simulink model "FlightSimulation"  (R2025a)
settings: Solver=ode4  StartTime=0.0  StopTime=Inf  FixedStep=time.dt  MaxStep=0.001  RelTol=1e-3
values from neighbouring files (symbols this model uses):
  AeroModel = init_IREC2025_CFDModel()    [RunSimulink.m]
  const = setupConstants()    [RunSimulink.m]
  kfConsts = getKfConsts()    [RunSimulink.m]
  kfErrInds = getErrorKfInds()    [RunSimulink.m]
  kfInds = getKfInds()    [RunSimulink.m]
  kfParams = initNavParams(kins)    [RunSimulink.m]
  kins = HPRC_RocketKinematics()    [RunSimulink.m]
  launchLLA = [launchLat, launchLon, launchAlt]    [RunSimulink.m]
  MotorModel = initMotorModel()    [RunSimulink.m]
  w_ib_x = 1e-10    [RunSimulink.m]
  w_ib_y = 1e-10    [RunSimulink.m]
  w_ib_z = 1e-10    [RunSimulink.m]
undefined symbols (not defined in the file or in its folder): Earth, F, fractalcoef, Light, MIL, Receive, Send, Sim3dSensor, simCfg, time, WGS84, WMM2020
libraries: simulink x6, aerolibatmos2 x5, aerolibfltsims x2, sim3dlib x2, aerolibsim3d x2, mspsensorlib x1, aerolibnav x1, aerolibgravity2 x1, aerolib6dof2 x1, aerolibwind2 x1, simulink_extras x1, matrix_library x1
(part 1 of 2)
settings Model: Creator=Blind  LastModifiedBy=Blind

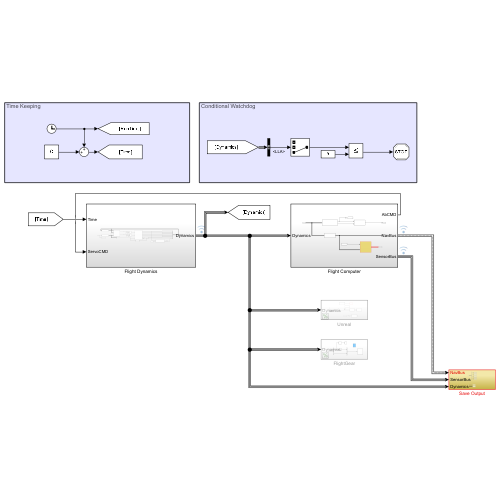
[thumbnail: Simulink's stored preview of the top-level diagram]
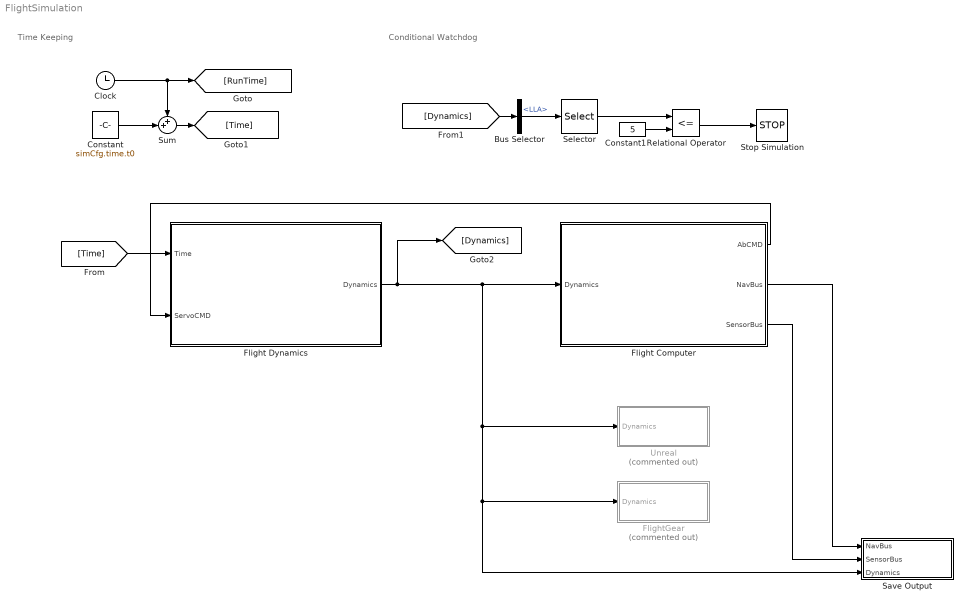
== system FlightSimulation ==
  note: Time Keeping
  note: Conditional Watchdog
  Bus Selector : BusSelector  OutputSignals=LLA
  Clock : Clock
  Constant : Constant  Value=simCfg.time.t0
  Constant1 : Constant  Value=5
  Flight Computer : Subsystem
  Flight Dynamics : Subsystem
  FlightGear : Subsystem  Commented=on
  Relational Operator : RelationalOperator  Operator=<=  OutDataTypeStr=boolean  RndMeth=Simplest  InputSameDT=off
  Save Output : Subsystem
  Selector : Selector  InputPortWidth=3  IndexOptions=Index vector (dialog)  Indices=3  OutputSizes=1
  Stop Simulation : Stop
  Sum : Sum  Inputs=++|
  Unreal : Subsystem  Commented=on
  wires:
  Clock/1 -> Sum/1, [RunTime]
  Constant/1 -> Sum/2
  Sum/1 -> [Time]
  [Time] -> Flight Dynamics/1(Time)
  Flight Dynamics/1(Dynamics) -> Flight Computer/1(Dynamics), Unreal/1(Dynamics), Save Output/3(Dynamics), FlightGear/1(Dynamics), [Dynamics]
  [Dynamics] -> Bus Selector/1
  Bus Selector/1 -> Selector/1  "<LLA>"
  Selector/1 -> Relational Operator/1
  Constant1/1 -> Relational Operator/2
  Relational Operator/1 -> Stop Simulation/1
  Flight Computer/1(AbCMD) -> Flight Dynamics/2(ServoCMD)
  Flight Computer/2(NavBus) -> Save Output/1(NavBus)
  Flight Computer/3(SensorBus) -> Save Output/2(SensorBus)

== system FlightSimulation/Flight Computer ==
  Dynamics : Inport
  Navigator : Subsystem  TreatAsAtomicUnit=on  SystemSampleTime=time.navDt
  Sensor Bus : Subsystem  TreatAsAtomicUnit=on
  State Machine : Subsystem
  Subsystem : Subsystem
  AbCMD : Outport
  NavBus : Outport  Port=2
  SensorBus : Outport  Port=3
  wires:
  Dynamics/1 -> Sensor Bus/1(Dynamics), State Machine/1(Dynamics)
  State Machine/1(State) -> [State], Subsystem/1(State)
  Subsystem/1(AbCMD) -> AbCMD/1
  State Machine/2(Guid) -> Subsystem/2(Guid)
  Sensor Bus/1(SensorBus) -> SensorBus/1, Navigator/2(SensorBus)
  Navigator/1(NavBus) -> NavBus/1
  [State] -> Navigator/1(State)

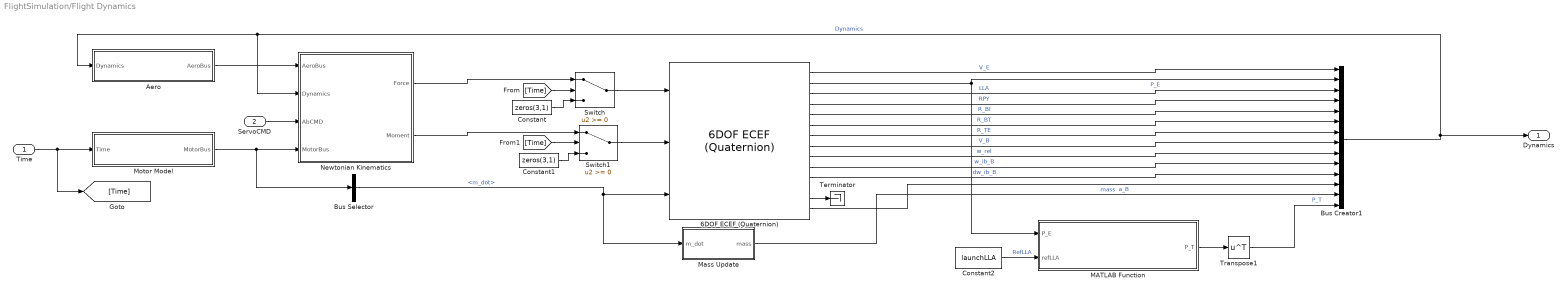
== system FlightSimulation/Flight Dynamics ==
  Time : Inport
  ServoCMD : Inport  Port=2
  6DOF ECEF (Quaternion) : aerolib6dof2/6DOF ECEF (Quaternion)  units=Metric (MKS)  mtype=Simple Variable  xg_0=launchLLA  Vm_0=V_0_B  eul_0=eul_0  pm_0=[w_ib_x; w_ib_y; w_ib_z]  mass_0=kins.m_0 + MotorModel.emptyWt + MotorModel.propWt  mass_e=kins.m_0 + MotorModel.emptyWt  mass_f=kins.m_0 + MotorModel.emptyWt + MotorModel.propWt  inertia=eye(3)  inertia_e=kins.I_empty  inertia_f=kins.I_full  vre_flag=off  abi_flag=on  ptype=Earth (WGS84)  R=6378137  F=1/298.257223563  w_E=7292115e-11  angle_in=Internal  LPM0=0  quat_statename=''  pm_statename=''  Vm_statename=''  posfixedframe_statename=''  posinertial_statename=''  LPM_statename=''  mass_statename=''
  Aero : Subsystem
  Bus Creator1 : BusCreator  Inputs=14
  Bus Selector : BusSelector  OutputSignals=m_dot
  Constant : Constant  Value=zeros(3,1)
  Constant1 : Constant  Value=zeros(3,1)
  Constant2 : Constant  Value=launchLLA
  MATLAB Function : MATLAB Function  TreatAsAtomicUnit=on
  Mass Update : Subsystem
  Motor Model : Subsystem
  Newtonian Kinematics : Subsystem
  Switch : Switch  SaturateOnIntegerOverflow=off  InputSameDT=off
  Switch1 : Switch  SaturateOnIntegerOverflow=off  InputSameDT=off
  Terminator : Terminator
  Transpose1 : Math  Operator=transpose
  Dynamics : Outport
  wires:
  Motor Model/1(MotorBus) -> Newtonian Kinematics/4(MotorBus), Bus Selector/1
  Time/1 -> [Time], Motor Model/1(Time)
  Bus Creator1/1 -> Newtonian Kinematics/2(Dynamics), Aero/1(Dynamics), Dynamics/1  "Dynamics"
  Aero/1(AeroBus) -> Newtonian Kinematics/1(AeroBus)
  Bus Selector/1 -> Mass Update/1(m_dot), 6DOF ECEF (Quaternion)/3  "<m_dot>"
  6DOF ECEF (Quaternion)/1 -> Bus Creator1/1  "V_E"
  6DOF ECEF (Quaternion)/2 -> MATLAB Function/1(P_E), Bus Creator1/2  "P_E"
  6DOF ECEF (Quaternion)/4 -> Bus Creator1/4  "RPY"
  6DOF ECEF (Quaternion)/5 -> Bus Creator1/5  "R_BI"
  6DOF ECEF (Quaternion)/6 -> Bus Creator1/6  "R_BT"
  6DOF ECEF (Quaternion)/7 -> Bus Creator1/7  "R_TE"
  6DOF ECEF (Quaternion)/8 -> Bus Creator1/8  "V_B"
  6DOF ECEF (Quaternion)/10 -> Bus Creator1/10  "w_ib_B"
  6DOF ECEF (Quaternion)/11 -> Bus Creator1/11  "dw_ib_B"
  Mass Update/1(mass) -> Bus Creator1/13  "mass"
  6DOF ECEF (Quaternion)/3 -> Bus Creator1/3  "LLA"
  6DOF ECEF (Quaternion)/9 -> Bus Creator1/9  "w_rel"
  Newtonian Kinematics/1(Force) -> Switch/1
  [Time] -> Switch/2
  Constant/1 -> Switch/3
  Switch/1 -> 6DOF ECEF (Quaternion)/1
  [Time] -> Switch1/2
  Constant1/1 -> Switch1/3
  Newtonian Kinematics/2(Moment) -> Switch1/1
  Switch1/1 -> 6DOF ECEF (Quaternion)/2
  6DOF ECEF (Quaternion)/13 -> Terminator/1
  ServoCMD/1 -> Newtonian Kinematics/3(AbCMD)
  6DOF ECEF (Quaternion)/14 -> Bus Creator1/12  "a_B"
  MATLAB Function/1(P_T) -> Transpose1/1
  Constant2/1 -> MATLAB Function/2(refLLA)  "RefLLA"
  Transpose1/1 -> Bus Creator1/14  "P_T"

== system FlightSimulation/FlightGear ==
  Dynamics : Inport
  Bus Selector : BusSelector  OutputSignals=LLA,RPY
  FlightGear Preconfigured 6DoF Animation : aerolibfltsims/FlightGear Preconfigured 6DoF Animation  xFlightGearVersion=v2019.1  DestinationIpAddress=127.0.0.1  DestinationPort=5502  SampleTime=1/30  packetVersion=24
  Generate Run Script : aerolibfltsims/Generate Run Script  Architecture=Mac  dataFlow=Send-Receive  GeometryModelName=HPMR  AirportId=KORH  RunwayId=29  InitialAltitude=7224  InitialHeading=113  OffsetDistance=4.72  OffsetAzimuth=0  InstallScenery=on  DisableShaders=on  OriginAddress=127.0.0.1  DestinationPort=5502  OriginPort=5505  LocalAddress=127.0.0.1  OutputFileName=runfg.sh  FlightGearBaseDirectory=/Applications/FlightGear.app
  Scope : Scope
      settings: ActiveDisplayYMinimum=2705.45233  ActiveDisplayYMaximum=2716.52751
  Selector : Selector  InputPortWidth=3  IndexOptions=Index vector (dialog)  Indices=[2 1 3]  OutputSizes=1
  Selector1 : Selector  InputPortWidth=3  IndexOptions=Index vector (dialog)  Indices=3  OutputSizes=1
  Vector Concatenate : Concatenate
  wires:
  Dynamics/1 -> Bus Selector/1
  Bus Selector/2 -> Vector Concatenate/2  "<RPY>"
  Vector Concatenate/1 -> FlightGear Preconfigured 6DoF Animation/1
  Bus Selector/1 -> Selector1/1, Selector/1  "<LLA>"
  Selector/1 -> Vector Concatenate/1
  Selector1/1 -> Scope/1

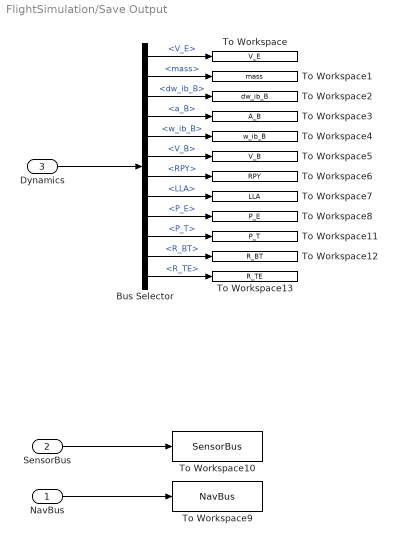
== system FlightSimulation/Save Output ==
  NavBus : Inport
  SensorBus : Inport  Port=2
  Dynamics : Inport  Port=3
  Bus Selector : BusSelector  OutputSignals=V_E,mass,dw_ib_B,a_B,w_ib_B,V_B,RPY,LLA,P_E,P_T,R_BT,R_TE
  To Workspace : ToWorkspace  VariableName=V_E  SaveFormat=Timeseries  SampleTime=-1
  To Workspace1 : ToWorkspace  VariableName=mass  SaveFormat=Timeseries  SampleTime=-1
  To Workspace10 : ToWorkspace  VariableName=SensorBus  SaveFormat=Timeseries  SampleTime=-1
  To Workspace11 : ToWorkspace  VariableName=P_T  SaveFormat=Timeseries  SampleTime=-1
  To Workspace12 : ToWorkspace  VariableName=R_BT  SaveFormat=Timeseries  SampleTime=-1
  To Workspace13 : ToWorkspace  VariableName=R_TE  SaveFormat=Timeseries  SampleTime=-1
  To Workspace2 : ToWorkspace  VariableName=dw_ib_B  SaveFormat=Timeseries  SampleTime=-1
  To Workspace3 : ToWorkspace  VariableName=A_B  SaveFormat=Timeseries  SampleTime=-1
  To Workspace4 : ToWorkspace  VariableName=w_ib_B  SaveFormat=Timeseries  SampleTime=-1
  To Workspace5 : ToWorkspace  VariableName=V_B  SaveFormat=Timeseries  SampleTime=-1
  To Workspace6 : ToWorkspace  VariableName=RPY  SaveFormat=Timeseries  SampleTime=-1
  To Workspace7 : ToWorkspace  VariableName=LLA  SaveFormat=Timeseries  SampleTime=-1
  To Workspace8 : ToWorkspace  VariableName=P_E  SaveFormat=Timeseries  SampleTime=-1
  To Workspace9 : ToWorkspace  VariableName=NavBus  SaveFormat=Timeseries  SampleTime=-1
  wires:
  Dynamics/1 -> Bus Selector/1
  Bus Selector/1 -> To Workspace/1  "<V_E>"
  Bus Selector/2 -> To Workspace1/1  "<mass>"
  Bus Selector/3 -> To Workspace2/1  "<dw_ib_B>"
  Bus Selector/4 -> To Workspace3/1  "<a_B>"
  Bus Selector/5 -> To Workspace4/1  "<w_ib_B>"
  Bus Selector/6 -> To Workspace5/1  "<V_B>"
  Bus Selector/7 -> To Workspace6/1  "<RPY>"
  Bus Selector/8 -> To Workspace7/1  "<LLA>"
  Bus Selector/9 -> To Workspace8/1  "<P_E>"
  NavBus/1 -> To Workspace9/1
  SensorBus/1 -> To Workspace10/1
  Bus Selector/10 -> To Workspace11/1  "<P_T>"
  Bus Selector/11 -> To Workspace12/1  "<R_BT>"
  Bus Selector/12 -> To Workspace13/1  "<R_TE>"

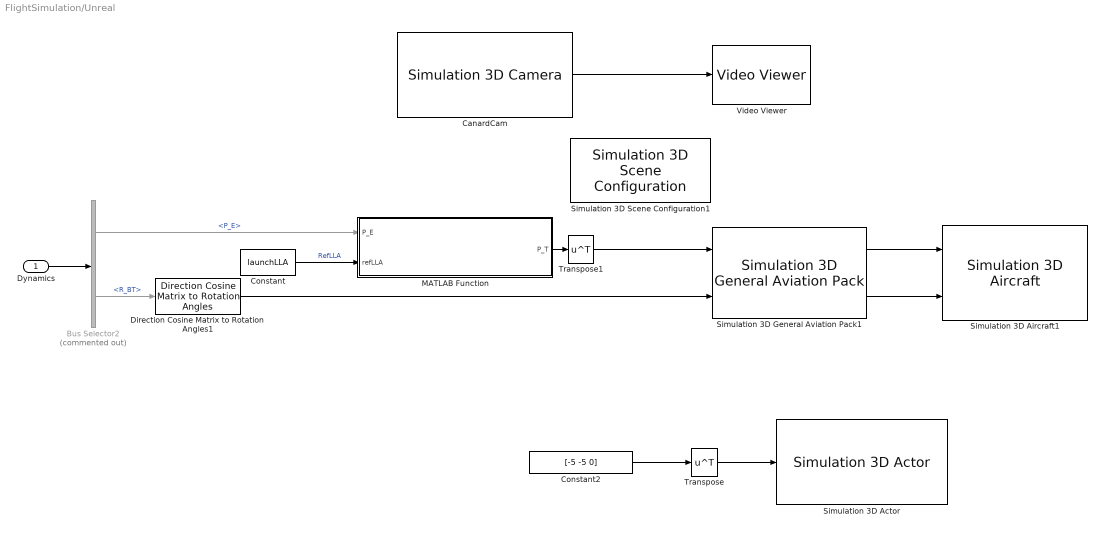
== system FlightSimulation/Unreal ==
  Dynamics : Inport
  Bus Selector2 : BusSelector  Commented=on  OutputSignals=P_E,R_BT
  CanardCam : sim3dcameralib/Simulation 3D Camera  Priority=1  sensorTag=Sim3dSensor�  sensorId=1  sensorName=Sim3dSensor�  vehTagList={'MissileNED';'Scene Origin';'Sim3dActor1'}  vehTag=MissileNED  CoordinateSystem=ISO8855  mountLoc=Origin  offsetFlag=on  tmountOffset=[1, 0.14, 0]  extTmount=off  rmountOffset=[0, 0, 180]  extRmount=off  FocalLength=[1109, 1109]  OpticalCenter=[640, 360]  ImageSize=[720, 1280]  RadialDistortion=[0, 0]  TangentialDistortion=[0, 0]  SensorSkew=0  VisualizeFieldOfView=off  FieldOfViewRange=61  DepthOutportEnabled=off  SemanticOutportEnabled=off  TransformOutportEnabled=off  SampleTime=-1  mountPoint=[1 0.14 0]  mountOrientation=[0 0 180]  aMode=4  ID=1
      settings: LibrarySourceBlock=uavsim3dlib/Simulation 3D Camera
  Constant : Constant  Value=launchLLA
  Constant2 : Constant  Value=[-5 -5 0]
  Direction Cosine Matrix to Rotation Angles1 : sharedtransform/Direction Cosine Matrix to Rotation Angles  rotationOrder=XYZ  aMode=aMode  action=None  tolerance=eps(2)
      settings: LibrarySourceBlock=|
      | aerolibtransform2/Direction Cosine Matrix
      | to Rotation Angles
  MATLAB Function : MATLAB Function  TreatAsAtomicUnit=on
  Simulation 3D Actor : sim3dlib/Simulation 3D Actor  Priority=1  ActorName=Sim3dActor1  ParentName=Scene Origin  Operation=Create at setup  InitScriptText=|  SampleTime=-1  Translation=[0 0 0]  Rotation=[0 0 0]  Scale=[1 1 1]  InputsText=Sim3dActor1.Translation  aMode=5  ActorTag=Sim3dActor1  ActorType=Sim3dActor  ID=1
      | % Reserved keywords:
      | % - Actor : handle to this actor object
      | % - World : handle to the world object
      | 
      | % Examples:
      | 
      | % Create a primitive geometry (optional)
      | % createShape(Actor, 'box', [1 1 1]);
      | 
      | % Initialize values (optional)
      | % Actor.Physics = true;
      | % Actor.Color = [1 0 0];
  Simulation 3D Aircraft1 : aerolibsim3d/Simulation 3D Aircraft  Priority=-1  Mesh=General aviation  MeshPath=/MathWorksAerospaceContent/Vehicles/Aircraft/Custom/Mesh/SK_HL20.SK_HL20  MeshPathAT=/MathWorksAerospaceContent/Vehicles/Aircraft/AirTransport/Mesh/SK_AirTransport.SK_AirTransport  MeshPathGA=/Game/Missile/MissileModel.MissileModel  AircraftColor=Red  ActorName=MissileNED  Translation=zeros(15, 3 )  Rotation=zeros(15, 3 )  ScaleInputPort=Dialog  Scale=[1 1 1]  InitialScale=[1 1 1]  IsGHSensorEnabled=off  AreGHRaysVisible=off  IsOutputReshapeEnabled=off  GHRayLength=1524  GHBodyOffset=0.90  GHFrontTireRadius=0.21  GHLeftTireRadius=0.21  GHRightTireRadius=0.21  WoWSensorTolerance=0.05  LightsConfig=Automatic lights  LandingLightIntensity=300000  LandingLightConeAngle=15  CustomLeftLandingLightLocation=[0 0 0]  CustomLeftLandingLightOrientation=[0 0 0]  CustomRightLandingLightLocation=[0 0 0]  CustomRightLandingLightOrientation=[0 0 0]  TaxiLightIntensity=150000  TaxiLightConeAngle=36  CustomTaxiLightLocation=[0 0 0]  CustomTaxiLightOrientation=[0 0 0]  NavLightIntensity=500  PositionLightIntensity=500  StrobeLightIntensity=5000  WingtipStrobePeriod=1.5  WingtipStrobePulseWidth=6  TailStrobePeriod=1.5  TailStrobePulseWidth=6  BeaconLightIntensity=4000  BeaconPeriod=1.5  BeaconPulseWidth=10  SampleTime=-1  ActorType=SimulinkVehicle  ID=C  aMode=0  ActorTag=MissileNED
  Simulation 3D General Aviation Pack1 : aerolibsim3d/Simulation 3D General Aviation Pack  Engine1_T=off  Engine1_R=off  Rudder_T=off  Rudder_R=off  Elevator_T=off  Elevator_R=off  Left_Aileron_T=off  Left_Aileron_R=off  Right_Aileron_T=off  Right_Aileron_R=off  Flaps_T=off  Flaps_R=off  Left_Spoiler_T=off  Left_Spoiler_R=off  Right_Spoiler_T=off  Right_Spoiler_R=off  Nose_Gear_T=off  Nose_Gear_R=off  Nose_Wheel_T=off  Nose_Wheel_R=off  Left_Gear_T=off  Left_Gear_R=off  Left_Wheel_T=off  Left_Wheel_R=off  Right_Gear_T=off  Right_Gear_R=off  Right_Wheel_T=off  Right_Wheel_R=off  GeoRadioButton=NED
      settings: AttributesFormatString=NED
  Simulation 3D Scene Configuration1 : sim3dlib/Simulation 3D Scene Configuration  Priority=0  ProjectFormat=Unreal Editor  SceneDesc=Airport  ProjectName=C:\Program Files\MATLAB\R2024b\toolbox\shared\sim3d_projects\automotive_project_windows\UE\WindowsNoEditor\VehicleSimulation.exe  ScenePath=/Game/Maps/HwStrght  UEProjPath=C:\Users\Blind\Workspace\FrostydevAvionics\Vanguard-FlightSim\AutoVrtlEnv\AutoVrtlEnv.uproject  EnableOpenDRIVE=off  vehTagList={'Custom';'MissileNED';'Scene Origin';'Sim3dActor1'}  vehTag=MissileNED  AttachedCameraRelativeTranslation=[0 0 0]  FreeCameraDefaultInitialTranslation=[-6, 0, 2]  AttachedCameraRelativeRotation=[0 0 0]  FreeCameraDefaultInitialRotation=[0, -15, 0]  ViewpointName=Custom  FreeCameraInitialTranslation=[-6, 0, 2]  ViewpointTranslation=[0 0 0]  FreeCameraInitialRotation=[0, -15, 0]  ViewpointRotation=[0 0 0]  OpVisEn=off  Ts=.02  EnableWindow=on  EnableRemoteAccess=off  EnableWeather=off  SunAzimuth=90  SunAltitude=40.0  EnableGeospatialSun=off  Latitude=0  Longitude=0  Date=2023-01-01  Time=10:30:00  GeoTimeZone=-5.0  SunDaylightSaving=off  wind=1  clouds=10  EnableVolumetricClouds=off  CloudCoverage=0  CloudAltitude=6  fog=0  rain=0  RaindropsEffect=off  SnowDensity=0  EnableGeospatial=off  TilesetSource=Earth terrain  UseTrueOrigin=off  OriginHeight=200  OriginLatitude=40.744652  OriginLongitude=-73.988864  MapStyle=Aerial  AdditionalAssetIDs=[]  UseAdvancedSunSky=off  SolarTime=11  TimeZone=-5  Day=21  Month=9  Year=2022  UseDaylightSavingTime=on  DSTStartDay=10  DSTStartMonth=3  DSTEndDay=3  DSTEndMonth=11  DSTSwitchHour=2  sensorTag=MainCamera2  sensorId=2  sensorName=MainCamera2  mountLoc=Origin  offsetFlag=off  tmountOffset=[0, 0, 0]  rmountOffset=[0, 0, 0]  HorizontalResolution=1280  VerticalResolution=720  HorizontalFOV=60  mountPoint=[0 0 0]  mountOrientation=[0 0 0]  aMode=0  ID=2  GeoTrigger=Inactive  ViewNameList={'Custom'}  ViewTranslationList={'[-6 0 2]'}  ViewRotationList={'[0 -15 0]'}
      settings: LibrarySourceBlock=aerolibsim3d/Simulation 3D Scene Configuration
  Transpose : Math  Operator=transpose
  Transpose1 : Math  Operator=transpose
  Video Viewer : VideoViewer  FigPos=[-1919 1151 1920 930]
  wires:
  CanardCam/1 -> Video Viewer/1
  Simulation 3D General Aviation Pack1/1 -> Simulation 3D Aircraft1/1
  Simulation 3D General Aviation Pack1/2 -> Simulation 3D Aircraft1/2
  Bus Selector2/1 -> MATLAB Function/1(P_E)  "<P_E>"
  Bus Selector2/2 -> Direction Cosine Matrix to Rotation Angles1/1  "<R_BT>"
  Direction Cosine Matrix to Rotation Angles1/1 -> Simulation 3D General Aviation Pack1/2
  Constant/1 -> MATLAB Function/2(refLLA)  "RefLLA"
  MATLAB Function/1(P_T) -> Transpose1/1
  Transpose1/1 -> Simulation 3D General Aviation Pack1/1
  Dynamics/1 -> Bus Selector2/1
  Constant2/1 -> Transpose/1
  Transpose/1 -> Simulation 3D Actor/1

== system FlightSimulation/Flight Computer/Navigator ==
  State : Inport
  SensorBus : Inport  Port=2
  Bus Selector2 : BusSelector  OutputSignals=ICM20948.sf_B_corr,ICM20948.w_ib_B_corr
  Compare To Constant1 : simulink/Logic and Bit Operations/Compare To Constant  relop===  const=1  OutDataTypeStr=boolean
  Delay One Step : Delay  DelayLength=1
  Delay One Step1 : Delay  DelayLength=1
  Delay1 : Delay  DelayLength=1  InitialConditionSource=Input port  InitialCondition=kfParams  ShowEnablePort=on  SampleTime=time.navDt
      settings: InputPortMap=u0,e6,p4
  Initialize Nav : Subsystem
  MATLAB Function : MATLAB Function  TreatAsAtomicUnit=on
  Update Step : Subsystem
  NavBus : Outport
  wires:
  SensorBus/1 -> Update Step/3(SensorBus), Bus Selector2/1, Initialize Nav/1(SensorBus)
  Initialize Nav/1(initFlag) -> Compare To Constant1/1
  Compare To Constant1/1 -> Update Step/Enable, Delay1/2
  Initialize Nav/2(NavBus) -> Delay1/3
  Delay1/1 -> MATLAB Function/1(navIn)  "NavBus"
  Bus Selector2/1 -> Delay One Step/1, MATLAB Function/2(sf_b)  "<sf_B_corr>"
  Bus Selector2/2 -> Delay One Step1/1, MATLAB Function/3(w_ib_b)  "<w_ib_B_corr>"
  MATLAB Function/1(navOut) -> Update Step/1(navBus)
  Update Step/1(navOut) -> Delay1/1, NavBus/1
  State/1 -> Update Step/2(State)
  Delay One Step/1 -> MATLAB Function/4(sf_b_prev)
  Delay One Step1/1 -> MATLAB Function/5(w_ib_b_prev)

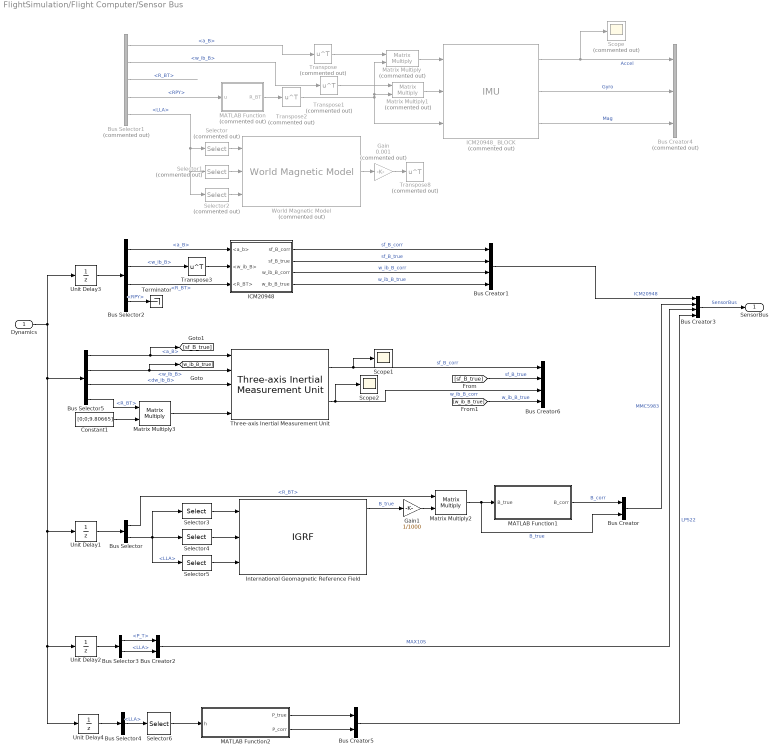
== system FlightSimulation/Flight Computer/Sensor Bus ==
  Dynamics : Inport
  Bus Creator : BusCreator  Inputs=2
  Bus Creator1 : BusCreator  Inputs=4
  Bus Creator2 : BusCreator  Inputs=2
  Bus Creator3 : BusCreator  Inputs=4
  Bus Creator4 : BusCreator  Commented=on  Inputs=3
  Bus Creator5 : BusCreator  Inputs=2
  Bus Creator6 : BusCreator  Inputs=4
  Bus Selector : BusSelector  OutputSignals=R_BT,LLA
  Bus Selector1 : BusSelector  Commented=on  OutputSignals=a_B,w_ib_B,R_BT,RPY,LLA
  Bus Selector2 : BusSelector  OutputSignals=a_B,w_ib_B,R_BT,RPY
  Bus Selector3 : BusSelector  OutputSignals=P_T,LLA
  Bus Selector4 : BusSelector  OutputSignals=LLA
  Bus Selector5 : BusSelector  OutputSignals=a_B,w_ib_B,dw_ib_B,R_BT
  Constant1 : Constant  Value=[0;0;9.80665]
  Gain : Gain  Commented=on  Gain=0.001
  Gain1 : Gain  Gain=1/1000
  ICM20948 : Subsystem
  ICM20948_ BLOCK : mspsensorlib/IMU  Commented=on  DispRefFrame=NED  TemperaturePort=off  Temperature=25  MagneticFieldPort=off  MagneticFieldNED=[19.9614, -4.8762, 47.062]  MagneticFieldENU=[ -2.4169, 27.5550, 16.0849 ]  SeedDouble=67  SimulateUsing=Interpreted execution  AccelParamsMeasurementRange=78.4532  AccelParamsResolution=0.0023958  AccelParamsConstantBias=[ 0, 0, 0 ]  AccelParamsAxesMisalignment=[ 100, 0, 0; 0, 100, 0; 0, 0, 100 ]  AccelParamsNoiseDensity=[ 0, 0, 0 ]  AccelParamsBiasInstability=[ 0, 0, 0 ]  AccelParamsBiasInstabilityNumerator=fractalcoef().Numerator  AccelParamsBiasInstabilityDenominator=fractalcoef().Denominator  AccelParamsRandomWalk=[0,0,0]  AccelParamsNoiseType=double-sided  AccelParamsTemperatureBias=[0,0,0]  AccelParamsTemperatureScaleFactor=[0,0,0]  GyroParamsMeasurementRange=100  GyroParamsResolution=0.0001332  GyroParamsConstantBias=[ 0, 0, 0 ]  GyroParamsAxesMisalignment=[ 100, 0, 0; 0, 100, 0; 0, 0, 100 ]  GyroParamsAccelerationBias=[ 0, 0, 0 ]  GyroParamsNoiseDensity=[ 0.00002618, 0.00002618, 0.00002618 ]  GyroParamsBiasInstability=[ 0, 0, 0 ]  GyroParamsBiasInstabilityNumerator=fractalcoef().Numerator  GyroParamsBiasInstabilityDenominator=fractalcoef().Denominator  GyroParamsRandomWalk=[ 0, 0, 0 ]  GyroParamsNoiseType=double-sided  GyroParamsTemperatureBias=[ 0.00087, 0.00087, 0.00087 ]  GyroParamsTemperatureScaleFactor=[ 0.03,0.03,0.03 ]  MagParamsMeasurementRange=4900  MagParamsResolution=0.15  MagParamsConstantBias=[ 0, 0, 0 ]  MagParamsAxesMisalignment=[ 100, 0, 0; 0, 100, 0; 0, 0, 100 ]  MagParamsNoiseDensity=[ 0, 0, 0 ]  MagParamsBiasInstability=[ 0, 0, 0 ]  MagParamsBiasInstabilityNumerator=fractalcoef().Numerator  MagParamsBiasInstabilityDenominator=fractalcoef().Denominator  MagParamsRandomWalk=[ 0, 0, 0 ]  MagParamsNoiseType=double-sided  MagParamsTemperatureBias=[ 0, 0, 0 ]  MagParamsTemperatureScaleFactor=[ 0, 0, 0 ]
  International Geomagnetic Reference Field : IGRF  time_in=off  month=January  day=1  sv_out=off
      settings: AttributesFormatString=%<generation>
  MATLAB Function : MATLAB Function  Commented=on  TreatAsAtomicUnit=on
  MATLAB Function1 : MATLAB Function  TreatAsAtomicUnit=on
  MATLAB Function2 : MATLAB Function  TreatAsAtomicUnit=on
  Matrix Multiply : Product  Commented=on  Multiplication=Matrix(*)
  Matrix Multiply1 : Product  Commented=on  Multiplication=Matrix(*)
  Matrix Multiply2 : Product  Multiplication=Matrix(*)
  Matrix Multiply3 : Product  Multiplication=Matrix(*)
  Scope : Scope  Commented=on
      settings: ActiveDisplayYMinimum=-91.1470131  ActiveDisplayYMaximum=35.7944499
  Scope1 : Scope
      settings: DataLoggingVariableName=ScopeData2
  Scope2 : Scope
      settings: ActiveDisplayYMinimum=-2.4796055057829047  ActiveDisplayYMaximum=2.7469070287295261  DataLoggingVariableName=ScopeData4
  Selector : Selector  Commented=on  InputPortWidth=3  IndexOptions=Index vector (dialog)  Indices=3  OutputSizes=1
  Selector1 : Selector  Commented=on  InputPortWidth=3  IndexOptions=Index vector (dialog)  Indices=1  OutputSizes=1
  Selector2 : Selector  Commented=on  InputPortWidth=3  IndexOptions=Index vector (dialog)  Indices=2  OutputSizes=1
  Selector3 : Selector  InputPortWidth=3  IndexOptions=Index vector (dialog)  Indices=3  OutputSizes=1
  Selector4 : Selector  InputPortWidth=3  IndexOptions=Index vector (dialog)  Indices=1  OutputSizes=1
  Selector5 : Selector  InputPortWidth=3  IndexOptions=Index vector (dialog)  Indices=1  OutputSizes=1
  Selector6 : Selector  InputPortWidth=3  IndexOptions=Index vector (dialog)  Indices=3  OutputSizes=1
  Terminator : Terminator
  Three-axis Inertial Measurement Unit : aerolibnav/Three-axis Inertial Measurement Unit  units=Metric (MKS)  imu=[0 0 0]  i_Ts=time.sensorDt  dtype_a=off  w_a=190  z_a=0.707  a_sf_cc=[1 0 0; 0 1 0; 0 0 1]  a_bias=[0 0 0]  a_sat="[-inf  -inf  -inf  inf inf inf]"  dtype_g=off  w_g=190  z_g=0.707  g_sf_cc=[1 0 0; 0 1 0; 0 0 1]  g_bias=[0 0 0]  g_sens=[0 0 0]  g_sat="[-inf  -inf  -inf  inf inf inf]"  i_rand=on  i_seeds=[23093 23094 23095 23096 23097 23098]  i_pow=[0.001 0.001 0.001 0.0001 0.0001 0.0001]
  Transpose{,1..2,8} (4 alike) : Math  Commented=on  Operator=transpose
  Transpose3 : Math  Operator=transpose
  Unit Delay{1..4} (4 alike) : UnitDelay  SampleTime=-1  HasFrameUpgradeWarning=on
  World Magnetic Model : aerolibgravity2/World Magnetic Model  Commented=on  model=WMM2020 (2020-2025)  customFile='WMM2020.COF'  units=Metric (MKS)  time_in=off  month=January  day=1  year=2020  action=Error  h_out=off  dec_out=off  inc_out=off  ti_out=off
  SensorBus : Outport
  wires:
  Dynamics/1 -> Unit Delay4/1, Unit Delay2/1, Unit Delay1/1, Bus Selector5/1, Unit Delay3/1
  Bus Creator3/1 -> SensorBus/1  "SensorBus"
  World Magnetic Model/1 -> Gain/1
  Selector/1 -> World Magnetic Model/1
  Selector1/1 -> World Magnetic Model/2
  Selector2/1 -> World Magnetic Model/3
  Unit Delay3/1 -> Bus Selector2/1
  Gain/1 -> Transpose8/1
  ICM20948_ BLOCK/2 -> Bus Creator4/2  "Gyro"
  ICM20948_ BLOCK/3 -> Bus Creator4/3  "Mag"
  Bus Selector1/5 -> Selector2/1, Selector1/1, Selector/1  "<LLA>"
  Bus Selector1/1 -> Transpose/1  "<a_B>"
  Bus Selector1/2 -> Transpose1/1  "<w_ib_B>"
  Bus Selector1/4 -> MATLAB Function/1(u)  "<RPY>"
  Matrix Multiply/1 -> ICM20948_ BLOCK/1
  Transpose/1 -> Matrix Multiply/1
  Matrix Multiply1/1 -> ICM20948_ BLOCK/2
  Transpose1/1 -> Matrix Multiply1/1
  MATLAB Function/1(R_BT) -> Transpose2/1
  Bus Selector1/3 -> ?  "<R_BT>"
  ICM20948_ BLOCK/1 -> Scope/1, Bus Creator4/1  "Accel"
  Transpose2/1 -> Matrix Multiply/2, Matrix Multiply1/2, ICM20948_ BLOCK/3
  Bus Selector2/1 -> ICM20948/1(<a_b>)  "<a_B>"
  Bus Selector2/2 -> Transpose3/1  "<w_ib_B>"
  Bus Selector2/4 -> Terminator/1  "<RPY>"
  Bus Selector2/3 -> ICM20948/3(<R_BT>)  "<R_BT>"
  ICM20948/1(sf_B_corr) -> Bus Creator1/1  "sf_B_corr"
  ICM20948/2(sf_B_true) -> Bus Creator1/2  "sf_B_true"
  ICM20948/3(w_ib_B_corr) -> Bus Creator1/3  "w_ib_B_corr"
  ICM20948/4(w_ib_B_true) -> Bus Creator1/4  "w_ib_B_true"
  Transpose3/1 -> ICM20948/2(<w_ib_B>)
  Unit Delay1/1 -> Bus Selector/1
  Selector3/1 -> International Geomagnetic Reference Field/1
  Bus Selector/2 -> Selector5/1, Selector3/1, Selector4/1  "<LLA>"
  Selector4/1 -> International Geomagnetic Reference Field/2
  Selector5/1 -> International Geomagnetic Reference Field/3
  MATLAB Function1/1(B_corr) -> Bus Creator/1  "B_corr"
  Bus Selector/1 -> Matrix Multiply2/1  "<R_BT>"
  Matrix Multiply2/1 -> Bus Creator/2, MATLAB Function1/1(B_true)  "B_true"
  International Geomagnetic Reference Field/1 -> Gain1/1  "B_true"
  Gain1/1 -> Matrix Multiply2/2
  Unit Delay2/1 -> Bus Selector3/1
  Bus Selector3/2 -> Bus Creator2/2  "<LLA>"
  Bus Selector3/1 -> Bus Creator2/1  "<P_T>"
  Unit Delay4/1 -> Bus Selector4/1
  Bus Selector4/1 -> Selector6/1  "<LLA>"
  Selector6/1 -> MATLAB Function2/1(h)
  MATLAB Function2/1(P_true) -> Bus Creator5/1
  MATLAB Function2/2(P_corr) -> Bus Creator5/2
  Bus Selector5/1 -> [sf_B_true], Three-axis Inertial Measurement Unit/1  "<a_B>"
  Bus Selector5/2 -> [w_ib_B_true], Three-axis Inertial Measurement Unit/2  "<w_ib_B>"
  Bus Selector5/3 -> Three-axis Inertial Measurement Unit/3  "<dw_ib_B>"
  Matrix Multiply3/1 -> Three-axis Inertial Measurement Unit/5
  Bus Selector5/4 -> Matrix Multiply3/1  "<R_BT>"
  Constant1/1 -> Matrix Multiply3/2
  Three-axis Inertial Measurement Unit/1 -> Scope1/1, Bus Creator6/1  "sf_B_corr"
  Three-axis Inertial Measurement Unit/2 -> Scope2/1, Bus Creator6/3  "w_ib_B_corr"
  [w_ib_B_true] -> Bus Creator6/4  "w_ib_B_true"
  [sf_B_true] -> Bus Creator6/2  "sf_B_true"
  Bus Creator/1 -> Bus Creator3/2  "MMC5983"
  Bus Creator2/1 -> Bus Creator3/3  "MAX10S"
  Bus Creator5/1 -> Bus Creator3/4  "LPS22"
  Bus Creator1/1 -> Bus Creator3/1  "ICM20948"

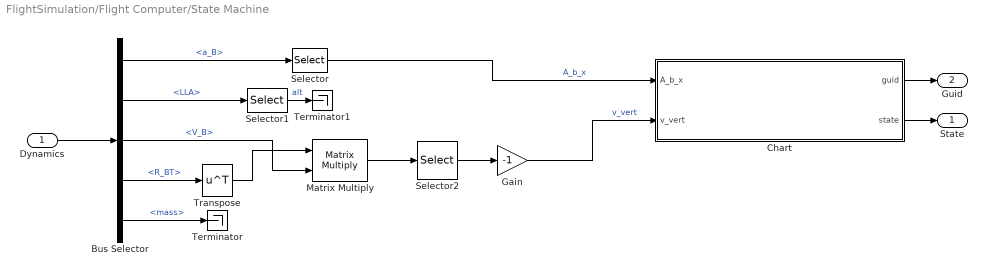
== system FlightSimulation/Flight Computer/State Machine ==
  Dynamics : Inport
  Bus Selector : BusSelector  OutputSignals=a_B,LLA,V_B,R_BT,mass
  Chart : Stateflow chart  TreatAsAtomicUnit=on
  Gain : Gain  Gain=-1
  Matrix Multiply : Product  Multiplication=Matrix(*)
  Selector : Selector  InputPortWidth=3  IndexOptions=Index vector (dialog)  Indices=1  OutputSizes=1
  Selector1 : Selector  InputPortWidth=3  IndexOptions=Index vector (dialog)  Indices=3  OutputSizes=1
  Selector2 : Selector  InputPortWidth=3  IndexOptions=Index vector (dialog)  Indices=3  OutputSizes=1
  Terminator : Terminator
  Terminator1 : Terminator
  Transpose : Math  Operator=transpose
  State : Outport
  Guid : Outport  Port=2
  wires:
  Matrix Multiply/1 -> Selector2/1
  Bus Selector/2 -> Selector1/1  "<LLA>"
  Bus Selector/3 -> Matrix Multiply/2  "<V_B>"
  Selector2/1 -> Gain/1
  Bus Selector/4 -> Transpose/1  "<R_BT>"
  Bus Selector/1 -> Selector/1  "<a_B>"
  Bus Selector/5 -> Terminator/1  "<mass>"
  Chart/2(state) -> State/1
  Dynamics/1 -> Bus Selector/1
  Chart/1(guid) -> Guid/1
  Selector/1 -> Chart/1(A_b_x)  "A_b_x"
  Gain/1 -> Chart/2(v_vert)  "v_vert"
  Transpose/1 -> Matrix Multiply/1
  Selector1/1 -> Terminator1/1  "alt"

== system FlightSimulation/Flight Computer/Subsystem ==
  State : Inport
  Guid : Inport  Port=2
  Compare To Constant : simulink/Logic and Bit Operations/Compare To Constant  relop===  const=1  OutDataTypeStr=boolean
  Constant : Constant  Value=0.75
  Constant1 : Constant  Value=0
  Switch1 : Switch  Criteria=u2 > Threshold  SaturateOnIntegerOverflow=off  InputSameDT=off
  Unit Delay : UnitDelay  SampleTime=-1  HasFrameUpgradeWarning=on
  AbCMD : Outport
  wires:
  Compare To Constant/1 -> Switch1/2
  Constant/1 -> Switch1/1
  Constant1/1 -> Switch1/3
  Switch1/1 -> AbCMD/1
  Unit Delay/1 -> Compare To Constant/1
  Guid/1 -> Unit Delay/1

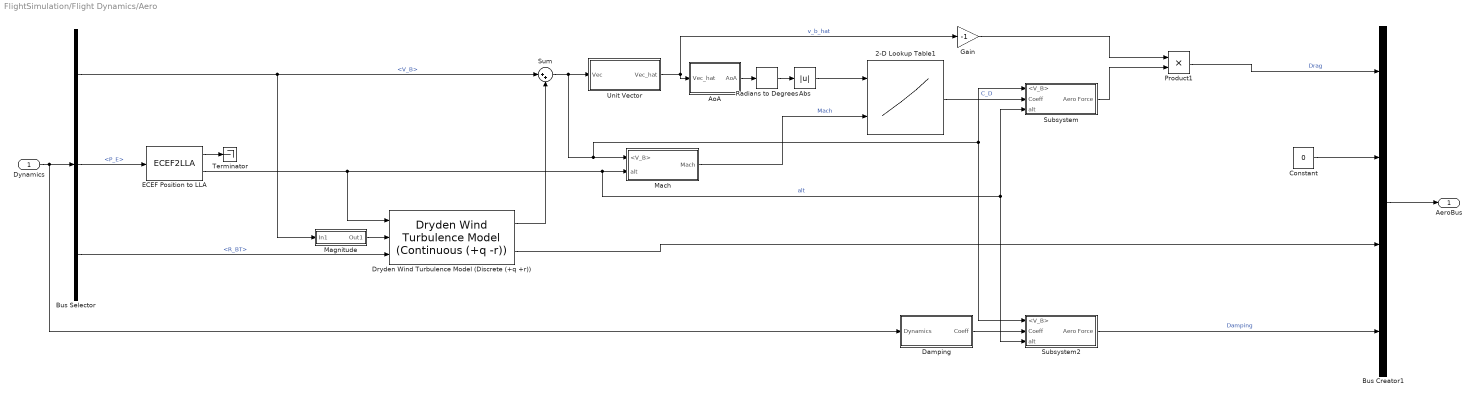
== system FlightSimulation/Flight Dynamics/Aero ==
  Dynamics : Inport
  2-D Lookup Table1 : Lookup_n-D  BreakpointsForDimension1=AeroModel.AoAs  BreakpointsForDimension2=AeroModel.MachNumbers  Table=AeroModel.CdGrid  ExtrapMethod=Clip  UseLastTableValue=on  ApplyAccurateEfficientRounding=on  InternalRulePriority=Speed  RndMeth=Simplest
      settings: InputPortMap=u0,u1
  Abs : Abs  SaturateOnIntegerOverflow=off
  AoA : Subsystem
  Bus Creator1 : BusCreator  Inputs=4
  Bus Selector : BusSelector  OutputSignals=V_B,P_E,R_BT
  Constant : Constant  Value=0
  Damping : Subsystem
  Dryden Wind Turbulence Model (Discrete (+q +r)) : aerolibwind2/Dryden Wind Turbulence Model  (Continuous (+q -r))  units=Metric (MKS)  spec=MIL-F-8785C  model=Discrete Dryden (+q +r)  W20=6  Wdeg=0  TurbProb=10^-2 - Light  L_high=533.4  Wingspan=0.127  ts=0.1  Seed=[23341 23342 23343 23344]  T_on=on
      settings: LibrarySourceBlock=|
      | aerolibwind2/Dryden Wind Turbulence Model
      | (Discrete (+q +r))
  ECEF Position to LLA : ECEF2LLA
  Gain : Gain  Gain=-1
  Mach : Subsystem
  Magnitude : Subsystem
  Product1 : Product
  Radians to Degrees : simulink_extras/Transformations/Radians to Degrees
  Subsystem : Subsystem
  Subsystem2 : Subsystem
  Sum : Sum  Inputs=|++
  Terminator : Terminator
  Unit Vector : Subsystem
  AeroBus : Outport
  wires:
  Dynamics/1 -> Damping/1(Dynamics), Bus Selector/1
  Bus Selector/2 -> ECEF Position to LLA/1  "<P_E>"
  ECEF Position to LLA/1 -> Terminator/1
  ECEF Position to LLA/2 -> Mach/2(alt), Subsystem/3(alt), Subsystem2/3(alt), Dryden Wind Turbulence Model (Discrete (+q +r))/1  "alt"
  Mach/1(Mach) -> 2-D Lookup Table1/2  "Mach"
  Unit Vector/1(Vec_hat) -> AoA/1(Vec_hat), Gain/1  "v_b_hat"
  AoA/1(AoA) -> Radians to Degrees/1
  Gain/1 -> Product1/1
  Product1/1 -> Bus Creator1/1  "Drag"
  Bus Creator1/1 -> AeroBus/1
  2-D Lookup Table1/1 -> Subsystem/2(Coeff)  "C_D"
  Subsystem/1(Aero Force) -> Product1/2
  Bus Selector/1 -> Magnitude/1(In1), Sum/1  "<V_B>"
  Magnitude/1(Out1) -> Dryden Wind Turbulence Model (Discrete (+q +r))/2
  Bus Selector/3 -> Dryden Wind Turbulence Model (Discrete (+q +r))/3  "<R_BT>"
  Sum/1 -> Subsystem/1(<V_B>), Subsystem2/1(<V_B>), Mach/1(<V_B>), Unit Vector/1(Vec)
  Dryden Wind Turbulence Model (Discrete (+q +r))/2 -> Bus Creator1/3
  Damping/1(Coeff) -> Subsystem2/2(Coeff)
  Subsystem2/1(Aero Force) -> Bus Creator1/4  "Damping"
  Dryden Wind Turbulence Model (Discrete (+q +r))/1 -> Sum/2
  Constant/1 -> Bus Creator1/2
  Radians to Degrees/1 -> Abs/1
  Abs/1 -> 2-D Lookup Table1/1

== system FlightSimulation/Flight Dynamics/Mass Update ==
  m_dot : Inport
  Constant : Constant  Value=kins.m_0 + MotorModel.emptyWt + MotorModel.propWt
  Integrator : Integrator
  Sum : Sum  Inputs=|-+
  mass : Outport
  wires:
  m_dot/1 -> Integrator/1
  Integrator/1 -> Sum/1
  Sum/1 -> mass/1
  Constant/1 -> Sum/2

== system FlightSimulation/Flight Dynamics/Motor Model ==
  Time : Inport
  2-D Lookup Table : Lookup_n-D  NumberOfTableDimensions=1  BreakpointsForDimension1=MotorModel.timePts  BreakpointsForDimension2=[1:3]  Table=MotorModel.thrustPts  ExtrapMethod=Clip  ApplyFullPrecisionForLinearInterpolation=on  InternalRulePriority=Speed  RndMeth=Simplest
  Bus Creator : BusCreator  Inputs=3
  Constant : Constant  Value=MotorModel.Isp
  Constant1 : Constant  Value=const.g_e
  Constant2 : Constant  Value=[1;0;0]
  Divide : Product  Inputs=*/
  Product : Product
  Product1 : Product
  MotorBus : Outport
  wires:
  Bus Creator/1 -> MotorBus/1
  Time/1 -> 2-D Lookup Table/1  "Time"
  Product/1 -> Bus Creator/3, Divide/2  "c"
  Constant/1 -> Product/1
  Constant1/1 -> Product/2
  Divide/1 -> Bus Creator/2  "m_dot"
  2-D Lookup Table/1 -> Divide/1, Product1/1  "Thrust"
  Constant2/1 -> Product1/2
  Product1/1 -> Bus Creator/1  "Thrust"

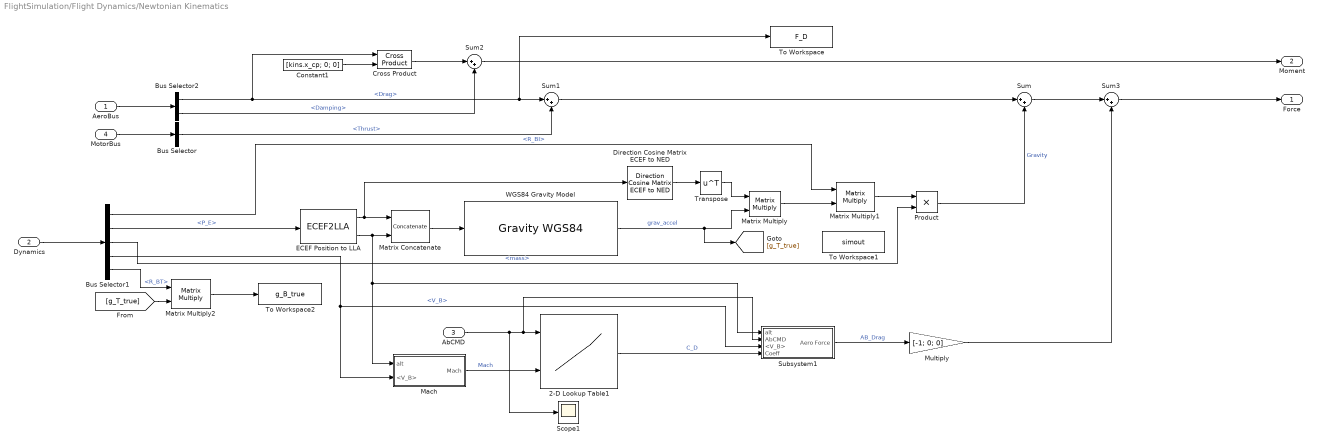
== system FlightSimulation/Flight Dynamics/Newtonian Kinematics ==
  AeroBus : Inport
  Dynamics : Inport  Port=2
  AbCMD : Inport  Port=3
  MotorBus : Inport  Port=4
  2-D Lookup Table1 : Lookup_n-D  BreakpointsForDimension1=AeroModel.AB.PercentActuation  BreakpointsForDimension2=AeroModel.AB.MachNumbers  Table=AeroModel.AB.CdGrid  InternalRulePriority=Speed  RndMeth=Simplest
      settings: InputPortMap=u0,u1
  Bus Selector : BusSelector  OutputSignals=Thrust
  Bus Selector1 : BusSelector  OutputSignals=R_BI,P_E,mass,V_B,R_BT
  Bus Selector2 : BusSelector  OutputSignals=Drag,Damping
  Constant1 : Constant  Value=[kins.x_cp; 0; 0]
  Cross Product : matrix_library/Cross Product
  Direction Cosine Matrix ECEF to NED : aerolibtransform2/Direction Cosine Matrix ECEF to NED
  ECEF Position to LLA : ECEF2LLA
  Mach : Subsystem
  Matrix Concatenate : Concatenate
  Matrix Multiply : Product  Multiplication=Matrix(*)
  Matrix Multiply1 : Product  Multiplication=Matrix(*)
  Matrix Multiply2 : Product  Multiplication=Matrix(*)
  Multiply : Gain  Gain=[-1; 0; 0]
  Product : Product
  Scope1 : Scope
      settings: ActiveDisplayYMinimum=-1  ActiveDisplayYMaximum=1  DataLoggingVariableName=ScopeData3
  Subsystem1 : Subsystem
  Sum{,1..3} (4 alike) : Sum  Inputs=|++
  To Workspace : ToWorkspace  VariableName=F_D  SaveFormat=Timeseries  SampleTime=-1
  To Workspace1 : ToWorkspace  VariableName=simout  SaveFormat=Timeseries  SampleTime=-1
  To Workspace2 : ToWorkspace  VariableName=g_B_true  SaveFormat=Timeseries  SampleTime=-1
  Transpose : Math  Operator=transpose
  "WGS84 Gravity Model  " : GravityWGS84
  Force : Outport
  Moment : Outport  Port=2
  wires:
  MotorBus/1 -> Bus Selector/1
  Dynamics/1 -> Bus Selector1/1
  AeroBus/1 -> Bus Selector2/1
  ECEF Position to LLA/1 -> Direction Cosine Matrix ECEF to NED/1, Matrix Concatenate/1
  ECEF Position to LLA/2 -> Subsystem1/1(alt), Mach/1(alt), Matrix Concatenate/2
  Matrix Concatenate/1 -> "WGS84 Gravity Model  "/1
  "WGS84 Gravity Model  "/1 -> [g_T_true], Matrix Multiply/2  "grav_accel"
  Direction Cosine Matrix ECEF to NED/1 -> Transpose/1
  Transpose/1 -> Matrix Multiply/1
  Sum1/1 -> Sum/1
  Bus Selector1/1 -> Matrix Multiply1/1  "<R_BI>"
  Bus Selector1/2 -> ECEF Position to LLA/1  "<P_E>"
  Bus Selector1/3 -> Product/2  "<mass>"
  Matrix Multiply/1 -> Matrix Multiply1/2
  Matrix Multiply1/1 -> Product/1
  Product/1 -> Sum/2  "Gravity"
  Bus Selector/1 -> Sum1/2  "<Thrust>"
  Bus Selector2/1 -> Cross Product/1, To Workspace/1, Sum1/1  "<Drag>"
  Bus Selector2/2 -> Sum2/2  "<Damping>"
  Cross Product/1 -> Sum2/1
  Constant1/1 -> Cross Product/2
  Sum2/1 -> Moment/1
  Bus Selector1/4 -> Mach/2(<V_B>), Subsystem1/3(<V_B>)  "<V_B>"
  2-D Lookup Table1/1 -> Subsystem1/4(Coeff)  "C_D"
  Subsystem1/1(Aero Force) -> Multiply/1  "AB_Drag"
  Sum/1 -> Sum3/1
  Bus Selector1/5 -> Matrix Multiply2/1  "<R_BT>"
  Sum3/1 -> Force/1
  Mach/1(Mach) -> 2-D Lookup Table1/2  "Mach"
  AbCMD/1 -> Scope1/1, Subsystem1/2(AbCMD), 2-D Lookup Table1/1
  Multiply/1 -> Sum3/2
  [g_T_true] -> Matrix Multiply2/2
  Matrix Multiply2/1 -> To Workspace2/1

== system FlightSimulation/Flight Computer/Navigator/Initialize Nav ==
  SensorBus : Inport
  Bus Creator : BusCreator  Inputs=6  OutDataTypeStr=Bus: kfParamsBus  NonVirtualBus=on
  Constant : Constant  Value=kfParams.f_pred
  Constant2 : Constant  Value=kfParams.Q_k
  Constant3 : Constant  Value=kfParams.P
  Constant4 : Constant  Value=kfParams.P_min
  Delay One Step : Delay  DelayLength=1
  Gain : Gain
  Initialize State : Subsystem
  initFlag : Outport
  NavBus : Outport  Port=2
  wires:
  SensorBus/1 -> Initialize State/2(SensorBus)
  Constant4/1 -> Bus Creator/5  "P_min"
  Constant3/1 -> Bus Creator/4  "P"
  Constant2/1 -> Bus Creator/3  "Q_k"
  Gain/1 -> Bus Creator/2  "x_pred"
  Initialize State/1(x_0) -> Gain/1, Bus Creator/1  "x"
  Bus Creator/1 -> NavBus/1
  Constant/1 -> Bus Creator/6  "f_pred"
  Initialize State/2(initFlag) -> Delay One Step/1, initFlag/1
  Delay One Step/1 -> Initialize State/1(initFlagLoop)

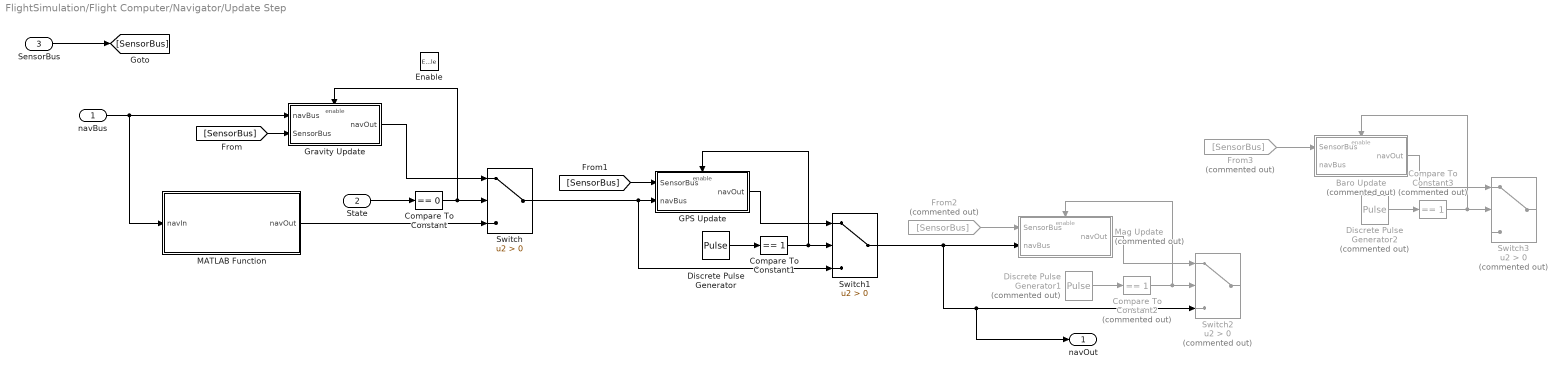
== system FlightSimulation/Flight Computer/Navigator/Update Step ==
  navBus : Inport
  State : Inport  Port=2
  SensorBus : Inport  Port=3
  Enable : EnablePort
  Baro Update : Subsystem  Commented=on  TreatAsAtomicUnit=on
  Compare To Constant : simulink/Logic and Bit Operations/Compare To Constant  relop===  const=0  OutDataTypeStr=boolean
  Compare To Constant1 : simulink/Logic and Bit Operations/Compare To Constant  relop===  const=1  OutDataTypeStr=boolean
  Compare To Constant2 : simulink/Logic and Bit Operations/Compare To Constant  Commented=on  relop===  const=1  OutDataTypeStr=boolean
  Compare To Constant3 : simulink/Logic and Bit Operations/Compare To Constant  Commented=on  relop===  const=1  OutDataTypeStr=boolean
  Discrete Pulse Generator : DiscretePulseGenerator  Period=5  SampleTime=time.navDt
  Discrete Pulse Generator1 : DiscretePulseGenerator  Commented=on  Period=5  SampleTime=time.navDt
  Discrete Pulse Generator2 : DiscretePulseGenerator  Commented=on  Amplitude=0  Period=5  SampleTime=time.navDt
  From2 : From  Commented=on  GotoTag=SensorBus
  From3 : From  Commented=on  GotoTag=SensorBus
  GPS Update : Subsystem  TreatAsAtomicUnit=on
  Gravity Update : Subsystem
  MATLAB Function : MATLAB Function  TreatAsAtomicUnit=on
  Mag Update : Subsystem  Commented=on  TreatAsAtomicUnit=on
  Switch : Switch  Criteria=u2 > Threshold  SaturateOnIntegerOverflow=off  InputSameDT=off
  Switch1 : Switch  Criteria=u2 > Threshold  SaturateOnIntegerOverflow=off  InputSameDT=off
  Switch2 : Switch  Commented=on  Criteria=u2 > Threshold  SaturateOnIntegerOverflow=off  InputSameDT=off
  Switch3 : Switch  Commented=on  Criteria=u2 > Threshold  SaturateOnIntegerOverflow=off  InputSameDT=off
  navOut : Outport
  wires:
  navBus/1 -> Gravity Update/1(navBus), MATLAB Function/1(navIn)
  Gravity Update/1(navOut) -> Switch/1
  Compare To Constant/1 -> Gravity Update/Enable, Switch/2
  MATLAB Function/1(navOut) -> Switch/3
  GPS Update/1(navOut) -> Switch1/1
  SensorBus/1 -> [SensorBus]
  [SensorBus] -> Gravity Update/2(SensorBus)
  Discrete Pulse Generator/1 -> Compare To Constant1/1
  Compare To Constant1/1 -> GPS Update/Enable, Switch1/2
  Compare To Constant2/1 -> Mag Update/Enable, Switch2/2
  Discrete Pulse Generator1/1 -> Compare To Constant2/1
  From2/1 -> Mag Update/1(SensorBus)
  Mag Update/1(navOut) -> Switch2/1
  Discrete Pulse Generator2/1 -> Compare To Constant3/1
  Baro Update/1(navOut) -> Switch3/1
  From3/1 -> Baro Update/1(SensorBus)
  Compare To Constant3/1 -> Baro Update/Enable, Switch3/2
  [SensorBus] -> GPS Update/1(SensorBus)
  Switch1/1 -> navOut/1, Switch2/3, Mag Update/2(navBus)
  Switch/1 -> Switch1/3, GPS Update/2(navBus)
  State/1 -> Compare To Constant/1

== system FlightSimulation/Flight Computer/Sensor Bus/ICM20948 ==
  <a_b> : Inport
  <w_ib_B> : Inport  Port=2
  <R_BT> : Inport  Port=3
  MATLAB Function : MATLAB Function  TreatAsAtomicUnit=on
  MATLAB Function 1 : MATLAB Function  TreatAsAtomicUnit=on
  MATLAB Function 2 : MATLAB Function  TreatAsAtomicUnit=on
  sf_B_corr : Outport
  sf_B_true : Outport  Port=2
  w_ib_B_corr : Outport  Port=3
  w_ib_B_true : Outport  Port=4
  wires:
  <a_b>/1 -> MATLAB Function/1(a_b)
  <R_BT>/1 -> MATLAB Function/2(R_BT)
  MATLAB Function/1(sf_true) -> sf_B_true/1, MATLAB Function 1/1(sf_true)
  MATLAB Function 1/1(sf_corr) -> sf_B_corr/1
  <w_ib_B>/1 -> MATLAB Function 2/1(gyro_true), w_ib_B_true/1
  MATLAB Function 2/1(gyro_corr) -> w_ib_B_corr/1

== system FlightSimulation/Flight Dynamics/Aero/AoA ==
  Vec_hat : Inport
  Atan : Trigonometry  Operator=atan
  Divide : Product  Inputs=*/
  Selector : Selector  InputPortWidth=3  IndexOptions=Index vector (dialog)  Indices=3  OutputSizes=1
  Selector1 : Selector  InputPortWidth=3  IndexOptions=Index vector (dialog)  Indices=1  OutputSizes=1
  AoA : Outport
  wires:
  Vec_hat/1 -> Selector1/1, Selector/1
  Selector/1 -> Divide/1
  Selector1/1 -> Divide/2
  Divide/1 -> Atan/1  "AoA"
  Atan/1 -> AoA/1

== system FlightSimulation/Flight Dynamics/Aero/Damping ==
  Dynamics : Inport
  Bus Selector : BusSelector  OutputSignals=w_ib_B
  Constant : Constant  Value=-AeroModel.damping.Cd_x*kins.S*kins.x_cp
  Constant1 : Constant  Value=-AeroModel.damping.Cd_y*kins.S*kins.x_cp
  Constant2 : Constant  Value=-AeroModel.damping.Cd_z*kins.S*kins.x_cp
  Product : Product
  Scope : Scope
      settings: ActiveDisplayYMinimum=-0.11753  ActiveDisplayYMaximum=0.06187  DataLoggingVariableName=ScopeData3
  Vector Concatenate : Concatenate  NumInputs=3
  Coeff : Outport
  wires:
  Constant/1 -> Vector Concatenate/1
  Constant1/1 -> Vector Concatenate/2
  Constant2/1 -> Vector Concatenate/3
  Dynamics/1 -> Bus Selector/1
  Bus Selector/1 -> Scope/1, Product/1  "<w_ib_B>"
  Vector Concatenate/1 -> Product/2
  Product/1 -> Coeff/1

== system FlightSimulation/Flight Dynamics/Aero/Mach ==
  <V_B> : Inport
  alt : Inport  Port=2
  Divide : Product  Inputs=*/
  Dot Product1 : DotProduct  OutDataTypeStr=Inherit: Inherit via internal rule
  ISA Atmosphere Model : aerolibatmos2/ISA Atmosphere Model  useExtended=off  action=Warning  custom=off  viscosityOut=off  g=9.80665  gamma=1.4  R=287.0531  L=0.0065  h_trop=11000  h_strat=20000  rho0=1.225  P0=101325  T0=288.15  h0=0  S=110.4  Tref=273.15  muref=1.716e-5
  Sqrt1 : Sqrt
  Terminator : Terminator
  Terminator1 : Terminator
  Terminator2 : Terminator
  Mach : Outport
  wires:
  Dot Product1/1 -> Sqrt1/1
  <V_B>/1 -> Dot Product1/2, Dot Product1/1
  Sqrt1/1 -> Divide/1  "v_B"
  alt/1 -> ISA Atmosphere Model/1
  ISA Atmosphere Model/2 -> Divide/2
  Divide/1 -> Mach/1
  ISA Atmosphere Model/1 -> Terminator/1
  ISA Atmosphere Model/3 -> Terminator1/1
  ISA Atmosphere Model/4 -> Terminator2/1

== system FlightSimulation/Flight Dynamics/Aero/Magnitude ==
  In1 : Inport
  Dot Product : DotProduct  OutDataTypeStr=Inherit: Inherit via internal rule
  Sqrt : Sqrt
  Out1 : Outport
  wires:
  In1/1 -> Dot Product/2, Dot Product/1
  Dot Product/1 -> Sqrt/1
  Sqrt/1 -> Out1/1

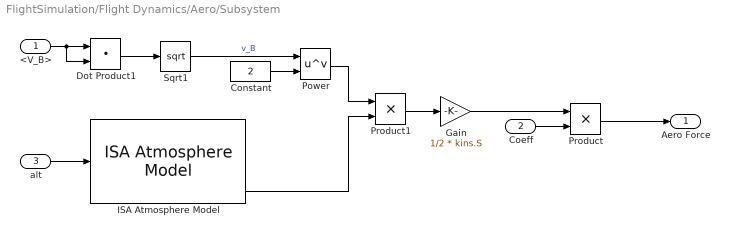
== system FlightSimulation/Flight Dynamics/Aero/Subsystem ==
  <V_B> : Inport
  Coeff : Inport  Port=2
  alt : Inport  Port=3
  Constant : Constant  Value=2
  Dot Product1 : DotProduct  OutDataTypeStr=Inherit: Inherit via internal rule
  Gain : Gain  Gain=1/2 * kins.S
  ISA Atmosphere Model : aerolibatmos2/ISA Atmosphere Model  useExtended=off  action=Warning  custom=off  viscosityOut=off  g=9.80665  gamma=1.4  R=287.0531  L=0.0065  h_trop=11000  h_strat=20000  rho0=1.225  P0=101325  T0=288.15  h0=0  S=110.4  Tref=273.15  muref=1.716e-5
  Power : Math  Operator=pow
  Product : Product
  Product1 : Product
  Sqrt1 : Sqrt
  Aero Force : Outport
  wires:
  alt/1 -> ISA Atmosphere Model/1
  ISA Atmosphere Model/4 -> Product1/2
  Dot Product1/1 -> Sqrt1/1
  <V_B>/1 -> Dot Product1/2, Dot Product1/1
  Product/1 -> Aero Force/1
  Coeff/1 -> Product/2
  Sqrt1/1 -> Power/1  "v_B"
  Constant/1 -> Power/2
  Power/1 -> Product1/1
  Product1/1 -> Gain/1
  Gain/1 -> Product/1

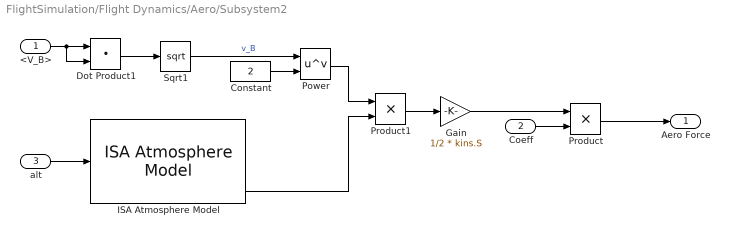
== system FlightSimulation/Flight Dynamics/Aero/Subsystem2 ==
  <V_B> : Inport
  Coeff : Inport  Port=2
  alt : Inport  Port=3
  Constant : Constant  Value=2
  Dot Product1 : DotProduct  OutDataTypeStr=Inherit: Inherit via internal rule
  Gain : Gain  Gain=1/2 * kins.S
  ISA Atmosphere Model : aerolibatmos2/ISA Atmosphere Model  useExtended=off  action=Warning  custom=off  viscosityOut=off  g=9.80665  gamma=1.4  R=287.0531  L=0.0065  h_trop=11000  h_strat=20000  rho0=1.225  P0=101325  T0=288.15  h0=0  S=110.4  Tref=273.15  muref=1.716e-5
  Power : Math  Operator=pow
  Product : Product
  Product1 : Product
  Sqrt1 : Sqrt
  Aero Force : Outport
  wires:
  alt/1 -> ISA Atmosphere Model/1
  ISA Atmosphere Model/4 -> Product1/2
  Dot Product1/1 -> Sqrt1/1
  <V_B>/1 -> Dot Product1/2, Dot Product1/1
  Product/1 -> Aero Force/1
  Coeff/1 -> Product/2
  Sqrt1/1 -> Power/1  "v_B"
  Constant/1 -> Power/2
  Power/1 -> Product1/1
  Product1/1 -> Gain/1
  Gain/1 -> Product/1

== system FlightSimulation/Flight Dynamics/Aero/Unit Vector ==
  Vec : Inport
  Divide : Product  Inputs=*/
  Dot Product1 : DotProduct  OutDataTypeStr=Inherit: Inherit via internal rule
  Sqrt1 : Sqrt
  Vec_hat : Outport
  wires:
  Vec/1 -> Divide/1, Dot Product1/2, Dot Product1/1
  Dot Product1/1 -> Sqrt1/1
  Sqrt1/1 -> Divide/2
  Divide/1 -> Vec_hat/1

== system FlightSimulation/Flight Dynamics/Newtonian Kinematics/Mach ==
  alt : Inport
  <V_B> : Inport  Port=2
  Divide : Product  Inputs=*/
  Dot Product1 : DotProduct  OutDataTypeStr=Inherit: Inherit via internal rule
  ISA Atmosphere Model : aerolibatmos2/ISA Atmosphere Model  useExtended=off  action=Warning  custom=off  viscosityOut=off  g=9.80665  gamma=1.4  R=287.0531  L=0.0065  h_trop=11000  h_strat=20000  rho0=1.225  P0=101325  T0=288.15  h0=0  S=110.4  Tref=273.15  muref=1.716e-5
  Sqrt1 : Sqrt
  Terminator : Terminator
  Terminator1 : Terminator
  Terminator2 : Terminator
  Mach : Outport
  wires:
  Dot Product1/1 -> Sqrt1/1
  <V_B>/1 -> Dot Product1/2, Dot Product1/1
  Sqrt1/1 -> Divide/1  "v_B"
  alt/1 -> ISA Atmosphere Model/1
  ISA Atmosphere Model/2 -> Divide/2
  Divide/1 -> Mach/1
  ISA Atmosphere Model/1 -> Terminator/1
  ISA Atmosphere Model/3 -> Terminator1/1
  ISA Atmosphere Model/4 -> Terminator2/1

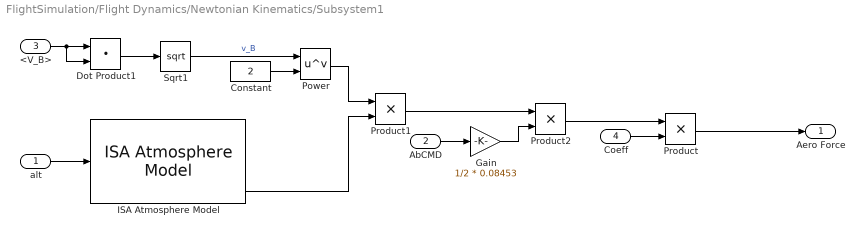
== system FlightSimulation/Flight Dynamics/Newtonian Kinematics/Subsystem1 ==
  alt : Inport
  AbCMD : Inport  Port=2
  <V_B> : Inport  Port=3
  Coeff : Inport  Port=4
  Constant : Constant  Value=2
  Dot Product1 : DotProduct  OutDataTypeStr=Inherit: Inherit via internal rule
  Gain : Gain  Gain=1/2 * 0.08453
  ISA Atmosphere Model : aerolibatmos2/ISA Atmosphere Model  useExtended=off  action=Warning  custom=off  viscosityOut=off  g=9.80665  gamma=1.4  R=287.0531  L=0.0065  h_trop=11000  h_strat=20000  rho0=1.225  P0=101325  T0=288.15  h0=0  S=110.4  Tref=273.15  muref=1.716e-5
  Power : Math  Operator=pow
  Product : Product
  Product1 : Product
  Product2 : Product
  Sqrt1 : Sqrt
  Aero Force : Outport
  wires:
  alt/1 -> ISA Atmosphere Model/1
  ISA Atmosphere Model/4 -> Product1/2
  Dot Product1/1 -> Sqrt1/1
  <V_B>/1 -> Dot Product1/2, Dot Product1/1
  Product/1 -> Aero Force/1
  Coeff/1 -> Product/2
  Sqrt1/1 -> Power/1  "v_B"
  Constant/1 -> Power/2
  Power/1 -> Product1/1
  AbCMD/1 -> Gain/1
  Product1/1 -> Product2/1
  Gain/1 -> Product2/2
  Product2/1 -> Product/1

== system FlightSimulation/Flight Computer/Navigator/Initialize Nav/Initialize State ==
  initFlagLoop : Inport
  SensorBus : Inport  Port=2
  Bus Selector2 : BusSelector  OutputSignals=ICM20948.sf_B_corr,MMC5983.B_corr
  MATLAB Function2 : MATLAB Function  TreatAsAtomicUnit=on
  MATLAB Function3 : MATLAB Function  TreatAsAtomicUnit=on
  x_0 : Outport
  initFlag : Outport  Port=2
  wires:
  SensorBus/1 -> Bus Selector2/1
  Bus Selector2/1 -> MATLAB Function2/1(a_b)  "<sf_B_corr>"
  Bus Selector2/2 -> MATLAB Function2/2(m_b)  "<B_corr>"
  MATLAB Function2/1(q_0) -> MATLAB Function3/2(q_0)  "q_0"
  MATLAB Function3/1(x_0) -> x_0/1
  MATLAB Function3/2(initFlag) -> initFlag/1
  initFlagLoop/1 -> MATLAB Function3/1(initFlagLoop)

== system FlightSimulation/Flight Computer/Navigator/Update Step/Baro Update ==
  SensorBus : Inport
  navBus : Inport  Port=2
  Enable : EnablePort
  Bus Selector : BusSelector  OutputSignals=LPS22.P_corr
  MATLAB Function : MATLAB Function  TreatAsAtomicUnit=on
  navOut : Outport
  wires:
  MATLAB Function/1(navOut) -> navOut/1
  navBus/1 -> MATLAB Function/1(navIn)
  SensorBus/1 -> Bus Selector/1
  Bus Selector/1 -> MATLAB Function/2(u_baro)  "<P_corr>"

== system FlightSimulation/Flight Computer/Navigator/Update Step/GPS Update ==
  SensorBus : Inport
  navBus : Inport  Port=2
  Enable : EnablePort
  Bus Selector : BusSelector  OutputSignals=MAX10S.P_T
  MATLAB Function : MATLAB Function  TreatAsAtomicUnit=on
  navOut : Outport
  wires:
  MATLAB Function/1(navOut) -> navOut/1
  navBus/1 -> MATLAB Function/1(navIn)
  SensorBus/1 -> Bus Selector/1
  Bus Selector/1 -> MATLAB Function/2(u_k)  "<P_T>"

== system FlightSimulation/Flight Computer/Navigator/Update Step/Gravity Update ==
  navBus : Inport
  SensorBus : Inport  Port=2
  Enable : EnablePort
  Bus Selector : BusSelector  OutputSignals=ICM20948.sf_B_corr
  MATLAB Function : MATLAB Function  TreatAsAtomicUnit=on
  navOut : Outport
  wires:
  navBus/1 -> MATLAB Function/1(navIn)
  SensorBus/1 -> Bus Selector/1
  Bus Selector/1 -> MATLAB Function/2(accelMeas)  "<sf_B_corr>"
  MATLAB Function/1(navOut) -> navOut/1

== system FlightSimulation/Flight Computer/Navigator/Update Step/Mag Update ==
  SensorBus : Inport
  navBus : Inport  Port=2
  Enable : EnablePort
  Bus Selector : BusSelector  OutputSignals=MMC5983.B_corr
  MATLAB Function : MATLAB Function  TreatAsAtomicUnit=on
  navOut : Outport
  wires:
  MATLAB Function/1(navOut) -> navOut/1
  navBus/1 -> MATLAB Function/1(navIn)
  SensorBus/1 -> Bus Selector/1
  Bus Selector/1 -> MATLAB Function/2(u_mag)  "<B_corr>"
